simulink model "SF013A_PullCmpActv"  (R2013b)
settings: Solver=FixedStepDiscrete  SolverMode=SingleTasking  StartTime=0.0  StopTime=1  FixedStep=0.002  RelTol=1e-3
values from neighbouring files (symbols this model uses):
  ARCHGLBPRM_100MILLISEC_SEC_F32 = DataDict.Constant    [SF013A_PullCmpActv_DataDict.m]
  ARCHGLBPRM_2MILLISEC_SEC_F32 = DataDict.Constant    [SF013A_PullCmpActv_DataDict.m]
  ARCHGLBPRM_FLOATZEROTHD_ULS_F32 = DataDict.Constant    [SF013A_PullCmpActv_DataDict.m]
  INTGTRSCARSHOTERM_ULS_F32 = DataDict.Constant    [SF013A_PullCmpActv_DataDict.m]
  LONGTERMINTGTRSCAR_ULS_F32 = DataDict.Constant    [SF013A_PullCmpActv_DataDict.m]
  MICROSECTOSEC_ULS_F32 = DataDict.Constant    [SF013A_PullCmpActv_DataDict.m]
  MINSTOSEC_SECPERMINS_F32 = DataDict.Constant    [SF013A_PullCmpActv_DataDict.m]
  PullCmpActvCmpLrnTiDecShoTerm = DataDict.Calibration    [SF013A_PullCmpActv_DataDict.m]
  PullCmpActvCmpLrnTiIncShoTerm = DataDict.Calibration    [SF013A_PullCmpActv_DataDict.m]
  PullCmpActvCmpLrnTiLongTerm = DataDict.Calibration    [SF013A_PullCmpActv_DataDict.m]
  PullCmpActvCmpShoTermRstHwAgThd = DataDict.Calibration    [SF013A_PullCmpActv_DataDict.m]
  PullCmpActvCmpShoTermRstHwTqThd = DataDict.Calibration    [SF013A_PullCmpActv_DataDict.m]
  PullCmpActvCmpShoTermRstLatAThd = DataDict.Calibration    [SF013A_PullCmpActv_DataDict.m]
  PullCmpActvCmpShoTermRstYawRateThd = DataDict.Calibration    [SF013A_PullCmpActv_DataDict.m]
  PullCmpActvEna = DataDict.Calibration    [SF013A_PullCmpActv_DataDict.m]
  PullCmpActvLongTermLim = DataDict.Calibration    [SF013A_PullCmpActv_DataDict.m]
  PullCmpActvLrngEnaAgConfMinMgn = DataDict.Calibration    [SF013A_PullCmpActv_DataDict.m]
  PullCmpActvLrngEnaHwAgMaxMgn = DataDict.Calibration    [SF013A_PullCmpActv_DataDict.m]
  PullCmpActvLrngEnaHwTqMaxMgn = DataDict.Calibration    [SF013A_PullCmpActv_DataDict.m]
  PullCmpActvLrngEnaHwVelMaxMgn = DataDict.Calibration    [SF013A_PullCmpActv_DataDict.m]
  PullCmpActvLrngEnaLatAMaxMgn = DataDict.Calibration    [SF013A_PullCmpActv_DataDict.m]
  PullCmpActvLrngEnaTiThd = DataDict.Calibration    [SF013A_PullCmpActv_DataDict.m]
  PullCmpActvLrngEnaVehSpdMaxMgn = DataDict.Calibration    [SF013A_PullCmpActv_DataDict.m]
  PullCmpActvLrngEnaVehSpdMinMgn = DataDict.Calibration    [SF013A_PullCmpActv_DataDict.m]
  PullCmpActvLrngEnaVehSpdRateMaxMgn = DataDict.Calibration    [SF013A_PullCmpActv_DataDict.m]
  PullCmpActvLrngEnaYawRateMaxMgn = DataDict.Calibration    [SF013A_PullCmpActv_DataDict.m]
  PullCmpActvOpstSignTiShoTerm = DataDict.Calibration    [SF013A_PullCmpActv_DataDict.m]
  PullCmpActvOutpMaxRate = DataDict.Calibration    [SF013A_PullCmpActv_DataDict.m]
  PullCmpActvPullCmpShoTermLim = DataDict.Calibration    [SF013A_PullCmpActv_DataDict.m]
  PullCmpActvPullCmpTotLim = DataDict.Calibration    [SF013A_PullCmpActv_DataDict.m]
  PullCmpActvPullErrLimLongTerm = DataDict.Calibration    [SF013A_PullCmpActv_DataDict.m]
  PullCmpActvPullErrMgnThd = DataDict.Calibration    [SF013A_PullCmpActv_DataDict.m]
  PullCmpActvPullErrShoTermLim = DataDict.Calibration    [SF013A_PullCmpActv_DataDict.m]
  PullCmpActvShoTermRampTi = DataDict.Calibration    [SF013A_PullCmpActv_DataDict.m]
  SysGlbPrmSysTqRat = DataDict.ImprtdCal    [SF013A_PullCmpActv_DataDict.m]
libraries: NxtrAbslt x9, Fil x8, NxtrLim x6, FixdToFloat x3, NxtrSign x3, NxtrMin x3, NxtrNvM x2, NxtrMax x2, simulink x1, FloatToFixd x1, LnrIntrpn x1
(part 2 of 3)

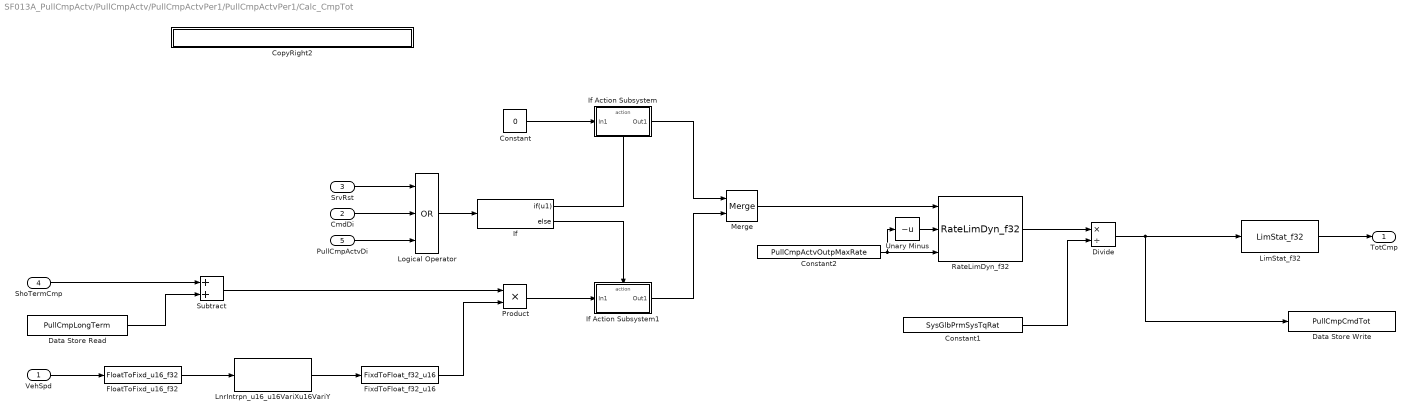
== system SF013A_PullCmpActv/PullCmpActv/PullCmpActvPer1/PullCmpActvPer1/Calc_CmpTot ==
  VehSpd : Inport
  CmdDi : Inport  Port=2
  SrvRst : Inport  Port=3
  ShoTermCmp : Inport  Port=4
  PullCmpActvDi : Inport  Port=5
  Constant : Constant  Value=0  OutDataTypeStr=single
  Constant1 : Constant  Value=SysGlbPrmSysTqRat
  Constant2 : Constant  Value=PullCmpActvOutpMaxRate
  CopyRight2 : Subsystem  Description=|  mask(Copyright Information){none=on}
      | Copyright info block.                                               
      |                                                                     
      | Place copyright information at the top of every subsystem in design.
      mask prompts: none "No parameters"
      mask help: Place copyright information at the top of every subsystem in design.
      mask Display:
      | NxtrConf = 'Nexteer Confidential';
      | 
      | sys = bdroot; %handle for the current model ("system")
      | first = get_param(sys,'Created');
      | if(isempty(first))
      |     first = datestr(now,'yyyy');
      | else
      |     first = first(end-3:end);  %year is last four digits
      | end
      | 
      | last = get_param(sys,'LastModifiedDate');
      | if isempty(last)
      |     last = datestr(now,'yyyy');
      | else
      |     last = last(end-3:end);
      | end
      | 
      | if strcmp(first,last)
      |     fprintf('%s -- Copyright %s Nexteer',NxtrConf,first)
      | else
      |     fprintf('%s -- %s%s- %s Nexteer',NxtrConf,char(169),first,last)
      | end
  Data Store Read : DataStoreRead  DataStoreName=PullCmpLongTerm
  Data Store Write : DataStoreWrite  DataStoreName=PullCmpCmdTot
  Divide : Product  Inputs=*/
  FixdToFloat_f32_u16 : FixdToFloat/FixdToFloat_f32_u16  Param1=14
  FloatToFixd_u16_f32 : FloatToFixd/FloatToFixd_u16_f32  Param1=7
  If : If  IfExpression=u1
  If Action Subsystem : Subsystem  TreatAsAtomicUnit=on
  If Action Subsystem1 : Subsystem  TreatAsAtomicUnit=on
  LimStat_f32 : NxtrLim/LimStat_f32  LoLim=SYSGLBPRM_MOTTQCMDLOLIM_MOTNWTMTR_F32  HiLim=SYSGLBPRM_MOTTQCMDHILIM_MOTNWTMTR_F32
      settings: AttributesFormatString=|
      | Low Limit: %<LoLim>
      | High Limit:%<HiLim>
  LnrIntrpn_u16_u16VariXu16VariY : LnrIntrpn/LnrIntrpn_u16_u16VariXu16VariY  XTbl=PullCmpActvVehSpdScaTblX  YTbl=PullCmpActvVehSpdScaTblY
      settings: AttributesFormatString=Lnr ( u16VariX , u16VariY )
  Logical Operator : Logic  Operator=OR  Inputs=3  AllPortsSameDT=off  OutDataTypeStr=boolean
  Merge : Merge
  Product : Product
  RateLimDyn_f32 : NxtrLim/RateLimDyn_f32  StVar=PullCmpCmdRateLimPrev  Ts=ARCHGLBPRM_2MILLISEC_SEC_F32
      settings: AttributesFormatString=StVar: %<StVar>
  Subtract : Sum
  Unary Minus : UnaryMinus
  TotCmp : Outport
  wires:
  SrvRst/1 -> Logical Operator/1
  CmdDi/1 -> Logical Operator/2
  ShoTermCmp/1 -> Subtract/1
  Data Store Read/1 -> Subtract/2
  FloatToFixd_u16_f32/1 -> LnrIntrpn_u16_u16VariXu16VariY/1
  VehSpd/1 -> FloatToFixd_u16_f32/1
  LnrIntrpn_u16_u16VariXu16VariY/1 -> FixdToFloat_f32_u16/1
  FixdToFloat_f32_u16/1 -> Product/2
  Subtract/1 -> Product/1
  Logical Operator/1 -> If/1
  Constant/1 -> If Action Subsystem/1(In1)
  Product/1 -> If Action Subsystem1/1(In1)
  RateLimDyn_f32/1 -> Divide/1
  Constant1/1 -> Divide/2
  Divide/1 -> Data Store Write/1, LimStat_f32/1
  Merge/1 -> RateLimDyn_f32/1
  If/1 -> If Action Subsystem/Action
  If Action Subsystem/1(Out1) -> Merge/1
  If/2 -> If Action Subsystem1/Action
  If Action Subsystem1/1(Out1) -> Merge/2
  Constant2/1 -> Unary Minus/1, RateLimDyn_f32/3
  Unary Minus/1 -> RateLimDyn_f32/2
  LimStat_f32/1 -> TotCmp/1
  PullCmpActvDi/1 -> Logical Operator/3

== system SF013A_PullCmpActv/PullCmpActv/PullCmpActvPer1/PullCmpActvPer1/CopyRight2 ==

== system SF013A_PullCmpActv/PullCmpActv/PullCmpActvPer1/PullCmpActvPer1/If RstPer1 == True set RstPer1 to False ==
  Action Port : ActionPort  ActionType=then
  Constant : Constant  Value=0  OutDataTypeStr=boolean
  Data Store Write1 : DataStoreWrite  DataStoreName=PullCmpShoTermRst
  wires:
  Constant/1 -> Data Store Write1/1

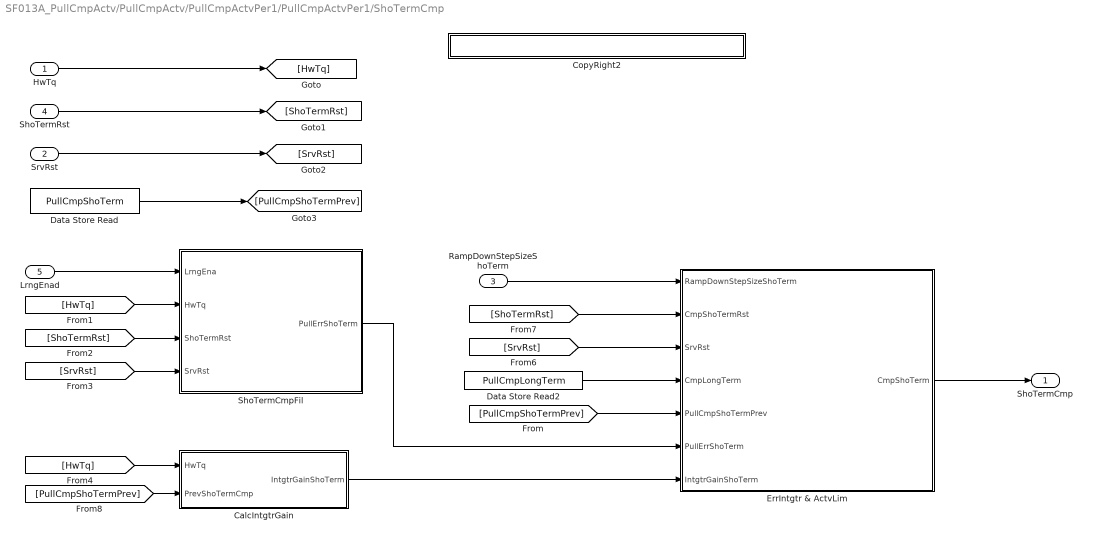
== system SF013A_PullCmpActv/PullCmpActv/PullCmpActvPer1/PullCmpActvPer1/ShoTermCmp ==
  "HwTq " : Inport
  SrvRst : Inport  Port=2
  RampDownStepSizeShoTerm : Inport  Port=3
  ShoTermRst : Inport  Port=4
  LrngEnad : Inport  Port=5
  "CalcIntgtrGain " : Subsystem  TreatAsAtomicUnit=on
  CopyRight2 : Subsystem  Description=|  mask(Copyright Information){none=on}
      | Copyright info block.                                               
      |                                                                     
      | Place copyright information at the top of every subsystem in design.
      mask prompts: none "No parameters"
      mask help: Place copyright information at the top of every subsystem in design.
      mask Display:
      | NxtrConf = 'Nexteer Confidential';
      | 
      | sys = bdroot; %handle for the current model ("system")
      | first = get_param(sys,'Created');
      | if(isempty(first))
      |     first = datestr(now,'yyyy');
      | else
      |     first = first(end-3:end);  %year is last four digits
      | end
      | 
      | last = get_param(sys,'LastModifiedDate');
      | if isempty(last)
      |     last = datestr(now,'yyyy');
      | else
      |     last = last(end-3:end);
      | end
      | 
      | if strcmp(first,last)
      |     fprintf('%s -- Copyright %s Nexteer',NxtrConf,first)
      | else
      |     fprintf('%s -- %s%s- %s Nexteer',NxtrConf,char(169),first,last)
      | end
  Data Store Read : DataStoreRead  DataStoreName=PullCmpShoTerm
  Data Store Read2 : DataStoreRead  DataStoreName=PullCmpLongTerm
  "ErrIntgtr & ActvLim " : Subsystem  TreatAsAtomicUnit=on
  ShoTermCmpFil : Subsystem  TreatAsAtomicUnit=on
  ShoTermCmp : Outport
  wires:
  "HwTq "/1 -> [HwTq]
  ShoTermRst/1 -> [ShoTermRst]
  SrvRst/1 -> [SrvRst]
  ShoTermCmpFil/1(PullErrShoTerm) -> "ErrIntgtr & ActvLim "/6(PullErrShoTerm)
  [HwTq] -> ShoTermCmpFil/2("HwTq ")
  LrngEnad/1 -> ShoTermCmpFil/1(LrngEna)
  [ShoTermRst] -> ShoTermCmpFil/3(ShoTermRst)
  [SrvRst] -> ShoTermCmpFil/4(SrvRst)
  [HwTq] -> "CalcIntgtrGain "/1("HwTq ")
  [PullCmpShoTermPrev] -> "CalcIntgtrGain "/2(PrevShoTermCmp)
  "CalcIntgtrGain "/1(IntgtrGainShoTerm) -> "ErrIntgtr & ActvLim "/7(IntgtrGainShoTerm)
  Data Store Read2/1 -> "ErrIntgtr & ActvLim "/4(CmpLongTerm)
  [PullCmpShoTermPrev] -> "ErrIntgtr & ActvLim "/5(PullCmpShoTermPrev)
  [SrvRst] -> "ErrIntgtr & ActvLim "/3("SrvRst ")
  [ShoTermRst] -> "ErrIntgtr & ActvLim "/2("CmpShoTermRst ")
  "ErrIntgtr & ActvLim "/1("CmpShoTerm ") -> ShoTermCmp/1
  Data Store Read/1 -> [PullCmpShoTermPrev]
  RampDownStepSizeShoTerm/1 -> "ErrIntgtr & ActvLim "/1(RampDownStepSizeShoTerm)

== system SF013A_PullCmpActv/PullCmpActv/PullCmpActvPer2/PullCmpActvPer2/CopyRight2 ==

== system SF013A_PullCmpActv/PullCmpActv/PullCmpActvPer2/PullCmpActvPer2/If PullCmpLongTermRst == True set PullCmpLongTermRst to False ==
  Action Port : ActionPort  ActionType=then
  Constant : Constant  Value=0  OutDataTypeStr=boolean
  CopyRight2 : Subsystem  Description=|  mask(Copyright Information){none=on}
      | Copyright info block.                                               
      |                                                                     
      | Place copyright information at the top of every subsystem in design.
      mask prompts: none "No parameters"
      mask help: Place copyright information at the top of every subsystem in design.
      mask Display:
      | NxtrConf = 'Nexteer Confidential';
      | 
      | sys = bdroot; %handle for the current model ("system")
      | first = get_param(sys,'Created');
      | if(isempty(first))
      |     first = datestr(now,'yyyy');
      | else
      |     first = first(end-3:end);  %year is last four digits
      | end
      | 
      | last = get_param(sys,'LastModifiedDate');
      | if isempty(last)
      |     last = datestr(now,'yyyy');
      | else
      |     last = last(end-3:end);
      | end
      | 
      | if strcmp(first,last)
      |     fprintf('%s -- Copyright %s Nexteer',NxtrConf,first)
      | else
      |     fprintf('%s -- %s%s- %s Nexteer',NxtrConf,char(169),first,last)
      | end
  Data Store Write1 : DataStoreWrite  DataStoreName=PullCmpLongTermRst
  wires:
  Constant/1 -> Data Store Write1/1

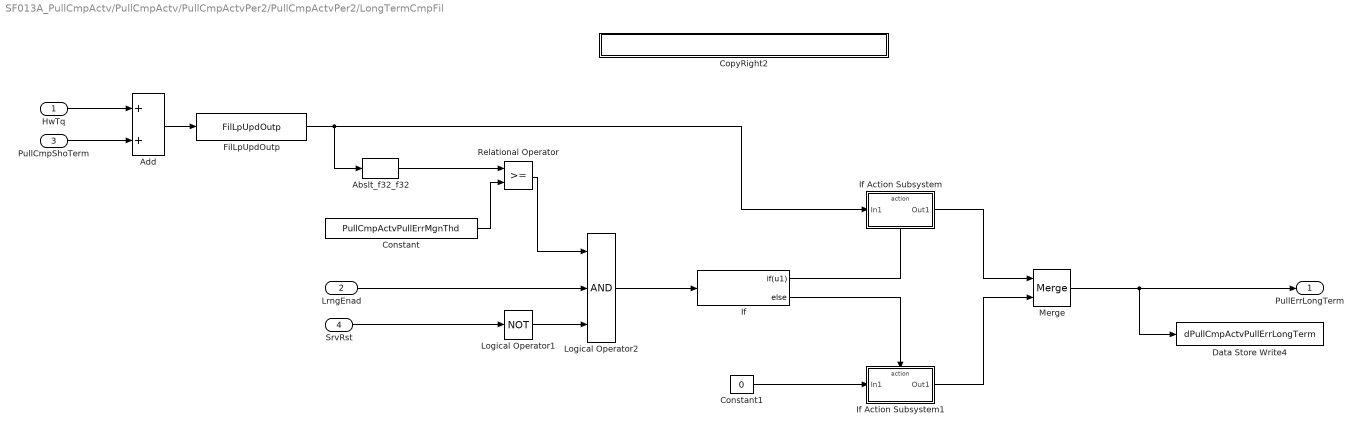
== system SF013A_PullCmpActv/PullCmpActv/PullCmpActvPer2/PullCmpActvPer2/LongTermCmpFil ==
  "HwTq " : Inport
  LrngEnad : Inport  Port=2
  PullCmpShoTerm : Inport  Port=3
  SrvRst : Inport  Port=4
  Abslt_f32_f32 : NxtrAbslt/Abslt_f32_f32  SFunctionSpec=single y1 = Abslt_f32_f32(single u1)
      settings: AttributesFormatString=%<Name>
  Add : Sum
  Constant : Constant  Value=PullCmpActvPullErrMgnThd
  Constant1 : Constant  Value=0  OutDataTypeStr=single
  CopyRight2 : Subsystem  Description=|  mask(Copyright Information){none=on}
      | Copyright info block.                                               
      |                                                                     
      | Place copyright information at the top of every subsystem in design.
      mask prompts: none "No parameters"
      mask help: Place copyright information at the top of every subsystem in design.
      mask Display:
      | NxtrConf = 'Nexteer Confidential';
      | 
      | sys = bdroot; %handle for the current model ("system")
      | first = get_param(sys,'Created');
      | if(isempty(first))
      |     first = datestr(now,'yyyy');
      | else
      |     first = first(end-3:end);  %year is last four digits
      | end
      | 
      | last = get_param(sys,'LastModifiedDate');
      | if isempty(last)
      |     last = datestr(now,'yyyy');
      | else
      |     last = last(end-3:end);
      | end
      | 
      | if strcmp(first,last)
      |     fprintf('%s -- Copyright %s Nexteer',NxtrConf,first)
      | else
      |     fprintf('%s -- %s%s- %s Nexteer',NxtrConf,char(169),first,last)
      | end
  Data Store Write4 : DataStoreWrite  DataStoreName=dPullCmpActvPullErrLongTerm
  FilLpUpdOutp : Fil/FilLpUpdOutp  StVar=HwTqLpFilLongTerm
      settings: AttributesFormatString=StVar: %<StVar>
  If : If  IfExpression=u1
  If Action Subsystem : Subsystem  TreatAsAtomicUnit=on
  If Action Subsystem1 : Subsystem  TreatAsAtomicUnit=on
  Logical Operator1 : Logic  Operator=NOT  Inputs=1  AllPortsSameDT=off  OutDataTypeStr=boolean
  Logical Operator2 : Logic  Inputs=3  AllPortsSameDT=off  OutDataTypeStr=boolean
  Merge : Merge
  Relational Operator : RelationalOperator  OutDataTypeStr=boolean
  PullErrLongTerm : Outport
  wires:
  FilLpUpdOutp/1 -> Abslt_f32_f32/1, If Action Subsystem/1(In1)
  Abslt_f32_f32/1 -> Relational Operator/1
  Constant/1 -> Relational Operator/2
  SrvRst/1 -> Logical Operator1/1
  Relational Operator/1 -> Logical Operator2/1
  LrngEnad/1 -> Logical Operator2/2
  Logical Operator1/1 -> Logical Operator2/3
  Constant1/1 -> If Action Subsystem1/1(In1)
  Merge/1 -> Data Store Write4/1, PullErrLongTerm/1
  Add/1 -> FilLpUpdOutp/1
  "HwTq "/1 -> Add/1
  PullCmpShoTerm/1 -> Add/2
  Logical Operator2/1 -> If/1
  If/1 -> If Action Subsystem/Action
  If/2 -> If Action Subsystem1/Action
  If Action Subsystem/1(Out1) -> Merge/1
  If Action Subsystem1/1(Out1) -> Merge/2

== system SF013A_PullCmpActv/PullCmpActv/PullCmpActvPer2/PullCmpActvPer2/LongTermErrIntgtr  ==
  "SrvRst " : Inport
  CmpLongTermPrev : Inport  Port=2
  PullErrLongTerm : Inport  Port=3
  Constant1 : Constant  Value=0  OutDataTypeStr=single
  CopyRight2 : Subsystem  Description=|  mask(Copyright Information){none=on}
      | Copyright info block.                                               
      |                                                                     
      | Place copyright information at the top of every subsystem in design.
      mask prompts: none "No parameters"
      mask help: Place copyright information at the top of every subsystem in design.
      mask Display:
      | NxtrConf = 'Nexteer Confidential';
      | 
      | sys = bdroot; %handle for the current model ("system")
      | first = get_param(sys,'Created');
      | if(isempty(first))
      |     first = datestr(now,'yyyy');
      | else
      |     first = first(end-3:end);  %year is last four digits
      | end
      | 
      | last = get_param(sys,'LastModifiedDate');
      | if isempty(last)
      |     last = datestr(now,'yyyy');
      | else
      |     last = last(end-3:end);
      | end
      | 
      | if strcmp(first,last)
      |     fprintf('%s -- Copyright %s Nexteer',NxtrConf,first)
      | else
      |     fprintf('%s -- %s%s- %s Nexteer',NxtrConf,char(169),first,last)
      | end
  Data Store Write2 : DataStoreWrite  DataStoreName=PullCmpLongTerm
  If : If  IfExpression=u1
  If Action Subsystem : Subsystem  TreatAsAtomicUnit=on
  If Action Subsystem1 : Subsystem  TreatAsAtomicUnit=on
  Merge : Merge
  wires:
  "SrvRst "/1 -> If/1
  Constant1/1 -> If Action Subsystem/1(In1)
  If/1 -> If Action Subsystem/Action
  If/2 -> If Action Subsystem1/Action
  Merge/1 -> Data Store Write2/1
  If Action Subsystem/1(Out1) -> Merge/1
  If Action Subsystem1/1(CmpLongTerm) -> Merge/2
  PullErrLongTerm/1 -> If Action Subsystem1/1(PullErrLongTerm)
  CmpLongTermPrev/1 -> If Action Subsystem1/2(CmpLongTermPrev)

== system SF013A_PullCmpActv/PullCmpActv/PullCmpActvPer1/PullCmpActvPer1/ActvCmpEna/CopyRight2 ==

== system SF013A_PullCmpActv/PullCmpActv/PullCmpActvPer1/PullCmpActvPer1/ActvCmpEna/ElapsedTime ==
  LrngEna : Inport
  Data Store Read : DataStoreRead  Priority=1  DataStoreName=LrngEnaPrev
      settings: AttributesFormatString="priority:  %<Priority>"
  Data Store Write : DataStoreWrite  Priority=2  DataStoreName=LrngEnaPrev
      settings: AttributesFormatString="priority:  %<Priority>"
  If : If  NumInputs=2  IfExpression=u1  ElseIfExpressions=u2
  If not true elapsed time = 0 : Subsystem  TreatAsAtomicUnit=on
  "If true and last step is true calculate elapsed time " : Subsystem  TreatAsAtomicUnit=on
  "If true and last step not true elapsed time = 0 get reference time " : Subsystem  TreatAsAtomicUnit=on
  Logical Operator : Logic  AllPortsSameDT=off  OutDataTypeStr=boolean
  Logical Operator1 : Logic  Operator=NOT  AllPortsSameDT=off  OutDataTypeStr=boolean
  Logical Operator2 : Logic  Operator=NOT  AllPortsSameDT=off  OutDataTypeStr=boolean
  Merge : Merge  Inputs=3
  ElapsedTime : Outport
  wires:
  If/1 -> If not true elapsed time = 0/Action
  If/2 -> "If true and last step not true elapsed time = 0 get reference time "/Action
  If/3 -> "If true and last step is true calculate elapsed time "/Action
  If not true elapsed time = 0/1(SpanTi) -> Merge/1
  "If true and last step not true elapsed time = 0 get reference time "/1("SpanTi ") -> Merge/2
  "If true and last step is true calculate elapsed time "/1(SpanTi) -> Merge/3
  Merge/1 -> ElapsedTime/1
  LrngEna/1 -> Logical Operator/1, Logical Operator2/1, Data Store Write/1
  Logical Operator1/1 -> Logical Operator/2
  Data Store Read/1 -> Logical Operator1/1
  Logical Operator/1 -> If/2
  Logical Operator2/1 -> If/1

== system SF013A_PullCmpActv/PullCmpActv/PullCmpActvPer1/PullCmpActvPer1/Calc_CmpTot/CopyRight2 ==

== system SF013A_PullCmpActv/PullCmpActv/PullCmpActvPer1/PullCmpActvPer1/Calc_CmpTot/If Action Subsystem ==
  In1 : Inport
  Action Port : ActionPort  ActionType=then
  CopyRight2 : Subsystem  Description=|  mask(Copyright Information){none=on}
      | Copyright info block.                                               
      |                                                                     
      | Place copyright information at the top of every subsystem in design.
      mask prompts: none "No parameters"
      mask help: Place copyright information at the top of every subsystem in design.
      mask Display:
      | NxtrConf = 'Nexteer Confidential';
      | 
      | sys = bdroot; %handle for the current model ("system")
      | first = get_param(sys,'Created');
      | if(isempty(first))
      |     first = datestr(now,'yyyy');
      | else
      |     first = first(end-3:end);  %year is last four digits
      | end
      | 
      | last = get_param(sys,'LastModifiedDate');
      | if isempty(last)
      |     last = datestr(now,'yyyy');
      | else
      |     last = last(end-3:end);
      | end
      | 
      | if strcmp(first,last)
      |     fprintf('%s -- Copyright %s Nexteer',NxtrConf,first)
      | else
      |     fprintf('%s -- %s%s- %s Nexteer',NxtrConf,char(169),first,last)
      | end
  Out1 : Outport
  wires:
  In1/1 -> Out1/1

== system SF013A_PullCmpActv/PullCmpActv/PullCmpActvPer1/PullCmpActvPer1/Calc_CmpTot/If Action Subsystem1 ==
  In1 : Inport
  Action Port : ActionPort  ActionType=else
  CopyRight2 : Subsystem  Description=|  mask(Copyright Information){none=on}
      | Copyright info block.                                               
      |                                                                     
      | Place copyright information at the top of every subsystem in design.
      mask prompts: none "No parameters"
      mask help: Place copyright information at the top of every subsystem in design.
      mask Display:
      | NxtrConf = 'Nexteer Confidential';
      | 
      | sys = bdroot; %handle for the current model ("system")
      | first = get_param(sys,'Created');
      | if(isempty(first))
      |     first = datestr(now,'yyyy');
      | else
      |     first = first(end-3:end);  %year is last four digits
      | end
      | 
      | last = get_param(sys,'LastModifiedDate');
      | if isempty(last)
      |     last = datestr(now,'yyyy');
      | else
      |     last = last(end-3:end);
      | end
      | 
      | if strcmp(first,last)
      |     fprintf('%s -- Copyright %s Nexteer',NxtrConf,first)
      | else
      |     fprintf('%s -- %s%s- %s Nexteer',NxtrConf,char(169),first,last)
      | end
  Out1 : Outport
  wires:
  In1/1 -> Out1/1

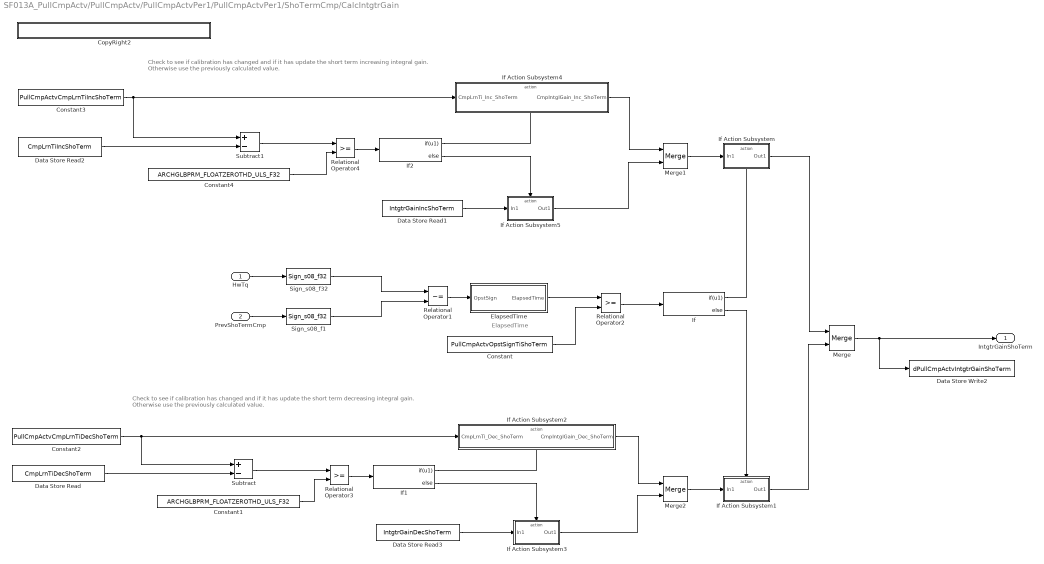
== system SF013A_PullCmpActv/PullCmpActv/PullCmpActvPer1/PullCmpActvPer1/ShoTermCmp/CalcIntgtrGain  ==
  note: Check to see if calibration has changed and if it has update the short term increasing integral gain.
      | Otherwise use the previously calculated value.
  note: ElapsedTime
  note: Check to see if calibration has changed and if it has update the short term decreasing integral gain.
      | Otherwise use the previously calculated value.
  "HwTq " : Inport
  PrevShoTermCmp : Inport  Port=2
  Constant : Constant  Value=PullCmpActvOpstSignTiShoTerm
  Constant1 : Constant  Value=ARCHGLBPRM_FLOATZEROTHD_ULS_F32
  Constant2 : Constant  Value=PullCmpActvCmpLrnTiDecShoTerm
  Constant3 : Constant  Value=PullCmpActvCmpLrnTiIncShoTerm
  Constant4 : Constant  Value=ARCHGLBPRM_FLOATZEROTHD_ULS_F32
  CopyRight2 : Subsystem  Description=|  mask(Copyright Information){none=on}
      | Copyright info block.                                               
      |                                                                     
      | Place copyright information at the top of every subsystem in design.
      mask prompts: none "No parameters"
      mask help: Place copyright information at the top of every subsystem in design.
      mask Display:
      | NxtrConf = 'Nexteer Confidential';
      | 
      | sys = bdroot; %handle for the current model ("system")
      | first = get_param(sys,'Created');
      | if(isempty(first))
      |     first = datestr(now,'yyyy');
      | else
      |     first = first(end-3:end);  %year is last four digits
      | end
      | 
      | last = get_param(sys,'LastModifiedDate');
      | if isempty(last)
      |     last = datestr(now,'yyyy');
      | else
      |     last = last(end-3:end);
      | end
      | 
      | if strcmp(first,last)
      |     fprintf('%s -- Copyright %s Nexteer',NxtrConf,first)
      | else
      |     fprintf('%s -- %s%s- %s Nexteer',NxtrConf,char(169),first,last)
      | end
  Data Store Read : DataStoreRead  DataStoreName=CmpLrnTiDecShoTerm
  Data Store Read1 : DataStoreRead  DataStoreName=IntgtrGainIncShoTerm
  Data Store Read2 : DataStoreRead  DataStoreName=CmpLrnTiIncShoTerm
  Data Store Read3 : DataStoreRead  DataStoreName=IntgtrGainDecShoTerm
  Data Store Write2 : DataStoreWrite  DataStoreName=dPullCmpActvIntgtrGainShoTerm
  ElapsedTime : Subsystem  TreatAsAtomicUnit=on
  If : If  IfExpression=u1
  If Action Subsystem : Subsystem  TreatAsAtomicUnit=on
  If Action Subsystem1 : Subsystem  TreatAsAtomicUnit=on
  If Action Subsystem2 : Subsystem  TreatAsAtomicUnit=on
  If Action Subsystem3 : Subsystem  TreatAsAtomicUnit=on
  If Action Subsystem4 : Subsystem  TreatAsAtomicUnit=on
  If Action Subsystem5 : Subsystem  TreatAsAtomicUnit=on
  If1 : If  IfExpression=u1
  If2 : If  IfExpression=u1
  Merge : Merge
  Merge1 : Merge
  Merge2 : Merge
  Relational Operator1 : RelationalOperator  Operator=~=  OutDataTypeStr=boolean
  Relational Operator2 : RelationalOperator  OutDataTypeStr=boolean
  Relational Operator3 : RelationalOperator  OutDataTypeStr=boolean
  Relational Operator4 : RelationalOperator  OutDataTypeStr=boolean
  Sign_s08_f1 : NxtrSign/Sign_s08_f32  SFunctionSpec=int8 y1 = Sign_s08_f32(single u1)
  Sign_s08_f32 : NxtrSign/Sign_s08_f32  SFunctionSpec=int8 y1 = Sign_s08_f32(single u1)
  Subtract : Sum  Inputs=+-
  Subtract1 : Sum  Inputs=+-
  IntgtrGainShoTerm : Outport
  wires:
  Relational Operator3/1 -> If1/1
  Data Store Read/1 -> Subtract/2
  If1/1 -> If Action Subsystem2/Action
  Constant2/1 -> Subtract/1, If Action Subsystem2/1(CmpLrnTi_Dec_ShoTerm)
  If2/1 -> If Action Subsystem4/Action
  Relational Operator4/1 -> If2/1
  Subtract/1 -> Relational Operator3/1
  Constant1/1 -> Relational Operator3/2
  Data Store Read2/1 -> Subtract1/2
  Constant3/1 -> If Action Subsystem4/1(CmpLrnTi_Inc_ShoTerm), Subtract1/1
  Subtract1/1 -> Relational Operator4/1
  Constant4/1 -> Relational Operator4/2
  "HwTq "/1 -> Sign_s08_f32/1
  PrevShoTermCmp/1 -> Sign_s08_f1/1
  Relational Operator1/1 -> ElapsedTime/1("OpstSign ")
  ElapsedTime/1(ElapsedTime) -> Relational Operator2/1
  Constant/1 -> Relational Operator2/2
  Merge/1 -> IntgtrGainShoTerm/1, Data Store Write2/1
  If/1 -> If Action Subsystem/Action
  If/2 -> If Action Subsystem1/Action
  Relational Operator2/1 -> If/1
  If Action Subsystem/1(Out1) -> Merge/1
  If Action Subsystem1/1(Out1) -> Merge/2
  Sign_s08_f32/1 -> Relational Operator1/1
  Sign_s08_f1/1 -> Relational Operator1/2
  If2/2 -> If Action Subsystem5/Action
  Data Store Read1/1 -> If Action Subsystem5/1(In1)
  If Action Subsystem5/1(Out1) -> Merge1/2
  If1/2 -> If Action Subsystem3/Action
  Data Store Read3/1 -> If Action Subsystem3/1(In1)
  If Action Subsystem4/1(CmpIntglGain_Inc_ShoTerm) -> Merge1/1
  Merge1/1 -> If Action Subsystem/1(In1)
  Merge2/1 -> If Action Subsystem1/1(In1)
  If Action Subsystem3/1(Out1) -> Merge2/2
  If Action Subsystem2/1(CmpIntglGain_Dec_ShoTerm) -> Merge2/1

== system SF013A_PullCmpActv/PullCmpActv/PullCmpActvPer1/PullCmpActvPer1/ShoTermCmp/CopyRight2 ==

== system SF013A_PullCmpActv/PullCmpActv/PullCmpActvPer1/PullCmpActvPer1/ShoTermCmp/ErrIntgtr & ActvLim  ==
  RampDownStepSizeShoTerm : Inport
  "CmpShoTermRst " : Inport  Port=2
  "SrvRst " : Inport  Port=3
  CmpLongTerm : Inport  Port=4
  PullCmpShoTermPrev : Inport  Port=5
  PullErrShoTerm : Inport  Port=6
  IntgtrGainShoTerm : Inport  Port=7
  Constant8 : Constant  Value=0  OutDataTypeStr=single
  CopyRight2 : Subsystem  Description=|  mask(Copyright Information){none=on}
      | Copyright info block.                                               
      |                                                                     
      | Place copyright information at the top of every subsystem in design.
      mask prompts: none "No parameters"
      mask help: Place copyright information at the top of every subsystem in design.
      mask Display:
      | NxtrConf = 'Nexteer Confidential';
      | 
      | sys = bdroot; %handle for the current model ("system")
      | first = get_param(sys,'Created');
      | if(isempty(first))
      |     first = datestr(now,'yyyy');
      | else
      |     first = first(end-3:end);  %year is last four digits
      | end
      | 
      | last = get_param(sys,'LastModifiedDate');
      | if isempty(last)
      |     last = datestr(now,'yyyy');
      | else
      |     last = last(end-3:end);
      | end
      | 
      | if strcmp(first,last)
      |     fprintf('%s -- Copyright %s Nexteer',NxtrConf,first)
      | else
      |     fprintf('%s -- %s%s- %s Nexteer',NxtrConf,char(169),first,last)
      | end
  Data Store Write : DataStoreWrite  DataStoreName=PullCmpShoTerm
  If Action Subsystem2 : Subsystem  TreatAsAtomicUnit=on
  If Action Subsystem3 : Subsystem  TreatAsAtomicUnit=on
  If1 : If  IfExpression=u1
  Merge : Merge
  "CmpShoTerm " : Outport
  wires:
  "CmpShoTermRst "/1 -> If Action Subsystem3/2("CmpShoTermRst ")
  RampDownStepSizeShoTerm/1 -> If Action Subsystem3/5(RampDownStepSizeShoTerm)
  If1/1 -> If Action Subsystem2/Action
  If1/2 -> If Action Subsystem3/Action
  PullErrShoTerm/1 -> If Action Subsystem3/1(PullErrShoTerm)
  CmpLongTerm/1 -> If Action Subsystem3/3(CmpLongTerm)
  IntgtrGainShoTerm/1 -> If Action Subsystem3/4(IntgtrGainShoTerm)
  Constant8/1 -> If Action Subsystem2/1(In1)
  "SrvRst "/1 -> If1/1
  If Action Subsystem2/1(Out1) -> Merge/1
  If Action Subsystem3/1(PullCmpShoTerm) -> Merge/2
  Merge/1 -> Data Store Write/1, "CmpShoTerm "/1
  PullCmpShoTermPrev/1 -> If Action Subsystem3/6(PullCmpShoTermPrev)

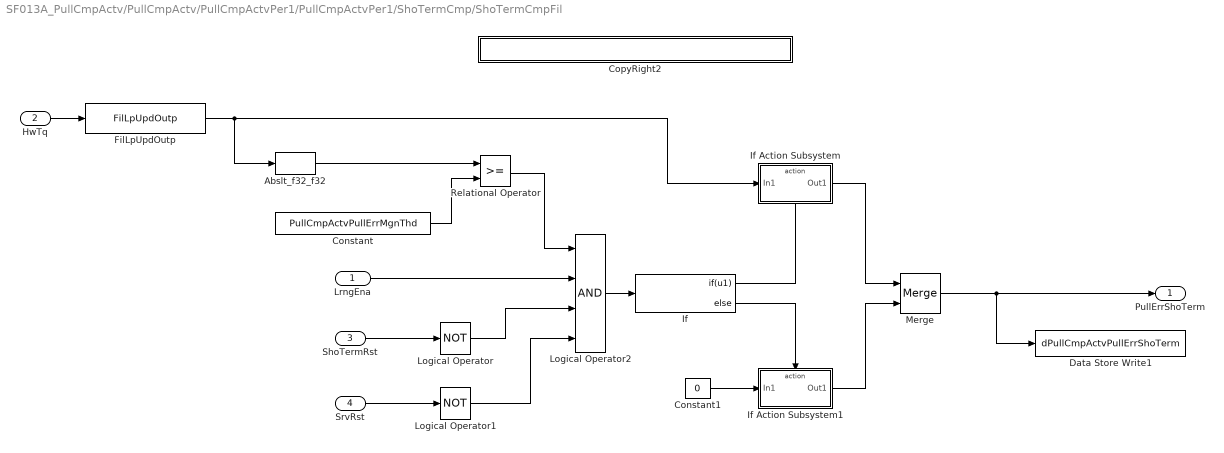
== system SF013A_PullCmpActv/PullCmpActv/PullCmpActvPer1/PullCmpActvPer1/ShoTermCmp/ShoTermCmpFil ==
  LrngEna : Inport
  "HwTq " : Inport  Port=2
  ShoTermRst : Inport  Port=3
  SrvRst : Inport  Port=4
  Abslt_f32_f32 : NxtrAbslt/Abslt_f32_f32  SFunctionSpec=single y1 = Abslt_f32_f32(single u1)
      settings: AttributesFormatString=%<Name>
  Constant : Constant  Value=PullCmpActvPullErrMgnThd
  Constant1 : Constant  Value=0  OutDataTypeStr=single
  CopyRight2 : Subsystem  Description=|  mask(Copyright Information){none=on}
      | Copyright info block.                                               
      |                                                                     
      | Place copyright information at the top of every subsystem in design.
      mask prompts: none "No parameters"
      mask help: Place copyright information at the top of every subsystem in design.
      mask Display:
      | NxtrConf = 'Nexteer Confidential';
      | 
      | sys = bdroot; %handle for the current model ("system")
      | first = get_param(sys,'Created');
      | if(isempty(first))
      |     first = datestr(now,'yyyy');
      | else
      |     first = first(end-3:end);  %year is last four digits
      | end
      | 
      | last = get_param(sys,'LastModifiedDate');
      | if isempty(last)
      |     last = datestr(now,'yyyy');
      | else
      |     last = last(end-3:end);
      | end
      | 
      | if strcmp(first,last)
      |     fprintf('%s -- Copyright %s Nexteer',NxtrConf,first)
      | else
      |     fprintf('%s -- %s%s- %s Nexteer',NxtrConf,char(169),first,last)
      | end
  Data Store Write1 : DataStoreWrite  DataStoreName=dPullCmpActvPullErrShoTerm
  FilLpUpdOutp : Fil/FilLpUpdOutp  StVar=HwTqLpFilShoTerm
      settings: AttributesFormatString=StVar: %<StVar>
  If : If  IfExpression=u1
  If Action Subsystem : Subsystem  TreatAsAtomicUnit=on
  If Action Subsystem1 : Subsystem  TreatAsAtomicUnit=on
  Logical Operator : Logic  Operator=NOT  Inputs=1  AllPortsSameDT=off  OutDataTypeStr=boolean
  Logical Operator1 : Logic  Operator=NOT  Inputs=1  AllPortsSameDT=off  OutDataTypeStr=boolean
  Logical Operator2 : Logic  Inputs=4  AllPortsSameDT=off  OutDataTypeStr=boolean
  Merge : Merge
  Relational Operator : RelationalOperator  OutDataTypeStr=boolean
  PullErrShoTerm : Outport
  wires:
  "HwTq "/1 -> FilLpUpdOutp/1
  FilLpUpdOutp/1 -> If Action Subsystem/1(In1), Abslt_f32_f32/1
  Abslt_f32_f32/1 -> Relational Operator/1
  Constant/1 -> Relational Operator/2
  SrvRst/1 -> Logical Operator1/1
  ShoTermRst/1 -> Logical Operator/1
  Relational Operator/1 -> Logical Operator2/1
  LrngEna/1 -> Logical Operator2/2
  Logical Operator/1 -> Logical Operator2/3
  Logical Operator1/1 -> Logical Operator2/4
  Logical Operator2/1 -> If/1
  Constant1/1 -> If Action Subsystem1/1(In1)
  Merge/1 -> Data Store Write1/1, PullErrShoTerm/1
  If/1 -> If Action Subsystem/Action
  If/2 -> If Action Subsystem1/Action
  If Action Subsystem/1(Out1) -> Merge/1
  If Action Subsystem1/1(Out1) -> Merge/2

== system SF013A_PullCmpActv/PullCmpActv/PullCmpActvPer2/PullCmpActvPer2/If PullCmpLongTermRst == True set PullCmpLongTermRst to False/CopyRight2 ==

== system SF013A_PullCmpActv/PullCmpActv/PullCmpActvPer2/PullCmpActvPer2/LongTermCmpFil/CopyRight2 ==

== system SF013A_PullCmpActv/PullCmpActv/PullCmpActvPer2/PullCmpActvPer2/LongTermCmpFil/If Action Subsystem ==
  In1 : Inport
  Action Port : ActionPort  ActionType=then
  CopyRight2 : Subsystem  Description=|  mask(Copyright Information){none=on}
      | Copyright info block.                                               
      |                                                                     
      | Place copyright information at the top of every subsystem in design.
      mask prompts: none "No parameters"
      mask help: Place copyright information at the top of every subsystem in design.
      mask Display:
      | NxtrConf = 'Nexteer Confidential';
      | 
      | sys = bdroot; %handle for the current model ("system")
      | first = get_param(sys,'Created');
      | if(isempty(first))
      |     first = datestr(now,'yyyy');
      | else
      |     first = first(end-3:end);  %year is last four digits
      | end
      | 
      | last = get_param(sys,'LastModifiedDate');
      | if isempty(last)
      |     last = datestr(now,'yyyy');
      | else
      |     last = last(end-3:end);
      | end
      | 
      | if strcmp(first,last)
      |     fprintf('%s -- Copyright %s Nexteer',NxtrConf,first)
      | else
      |     fprintf('%s -- %s%s- %s Nexteer',NxtrConf,char(169),first,last)
      | end
  Out1 : Outport
  wires:
  In1/1 -> Out1/1

== system SF013A_PullCmpActv/PullCmpActv/PullCmpActvPer2/PullCmpActvPer2/LongTermCmpFil/If Action Subsystem1 ==
  In1 : Inport
  Action Port : ActionPort  ActionType=else
  CopyRight2 : Subsystem  Description=|  mask(Copyright Information){none=on}
      | Copyright info block.                                               
      |                                                                     
      | Place copyright information at the top of every subsystem in design.
      mask prompts: none "No parameters"
      mask help: Place copyright information at the top of every subsystem in design.
      mask Display:
      | NxtrConf = 'Nexteer Confidential';
      | 
      | sys = bdroot; %handle for the current model ("system")
      | first = get_param(sys,'Created');
      | if(isempty(first))
      |     first = datestr(now,'yyyy');
      | else
      |     first = first(end-3:end);  %year is last four digits
      | end
      | 
      | last = get_param(sys,'LastModifiedDate');
      | if isempty(last)
      |     last = datestr(now,'yyyy');
      | else
      |     last = last(end-3:end);
      | end
      | 
      | if strcmp(first,last)
      |     fprintf('%s -- Copyright %s Nexteer',NxtrConf,first)
      | else
      |     fprintf('%s -- %s%s- %s Nexteer',NxtrConf,char(169),first,last)
      | end
  Out1 : Outport
  wires:
  In1/1 -> Out1/1

== system SF013A_PullCmpActv/PullCmpActv/PullCmpActvPer2/PullCmpActvPer2/LongTermErrIntgtr /CopyRight2 ==

== system SF013A_PullCmpActv/PullCmpActv/PullCmpActvPer2/PullCmpActvPer2/LongTermErrIntgtr /If Action Subsystem ==
  In1 : Inport
  Action Port : ActionPort  ActionType=then
  CopyRight2 : Subsystem  Description=|  mask(Copyright Information){none=on}
      | Copyright info block.                                               
      |                                                                     
      | Place copyright information at the top of every subsystem in design.
      mask prompts: none "No parameters"
      mask help: Place copyright information at the top of every subsystem in design.
      mask Display:
      | NxtrConf = 'Nexteer Confidential';
      | 
      | sys = bdroot; %handle for the current model ("system")
      | first = get_param(sys,'Created');
      | if(isempty(first))
      |     first = datestr(now,'yyyy');
      | else
      |     first = first(end-3:end);  %year is last four digits
      | end
      | 
      | last = get_param(sys,'LastModifiedDate');
      | if isempty(last)
      |     last = datestr(now,'yyyy');
      | else
      |     last = last(end-3:end);
      | end
      | 
      | if strcmp(first,last)
      |     fprintf('%s -- Copyright %s Nexteer',NxtrConf,first)
      | else
      |     fprintf('%s -- %s%s- %s Nexteer',NxtrConf,char(169),first,last)
      | end
  Out1 : Outport
  wires:
  In1/1 -> Out1/1

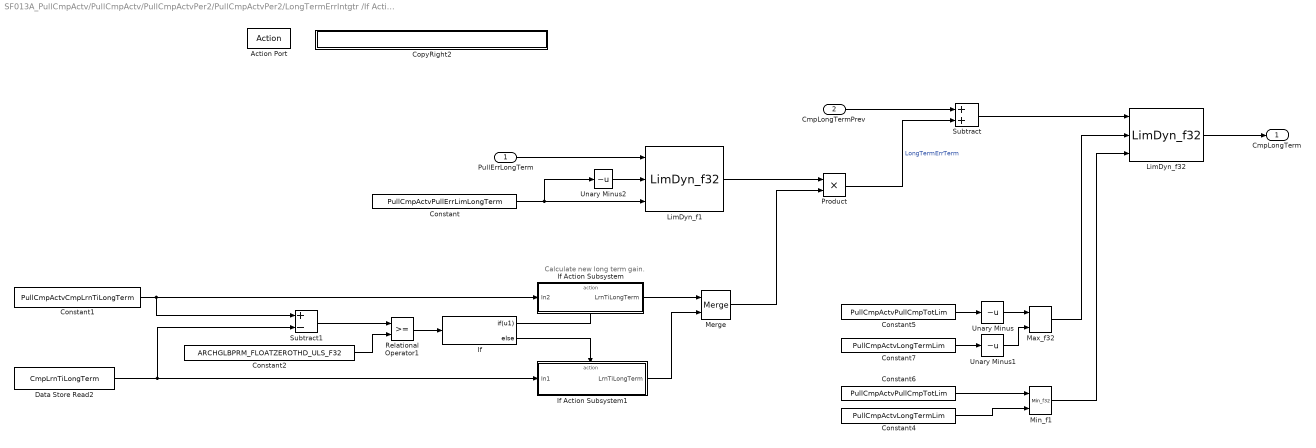
== system SF013A_PullCmpActv/PullCmpActv/PullCmpActvPer2/PullCmpActvPer2/LongTermErrIntgtr /If Action Subsystem1 ==
  note: Calculate new long term gain.
  PullErrLongTerm : Inport
  CmpLongTermPrev : Inport  Port=2
  Action Port : ActionPort  ActionType=else
  Constant : Constant  Value=PullCmpActvPullErrLimLongTerm
  Constant1 : Constant  Value=PullCmpActvCmpLrnTiLongTerm
  Constant2 : Constant  Value=ARCHGLBPRM_FLOATZEROTHD_ULS_F32
  Constant4 : Constant  Value=PullCmpActvLongTermLim
  Constant5 : Constant  Value=PullCmpActvPullCmpTotLim
  Constant6 : Constant  Value=PullCmpActvPullCmpTotLim
  Constant7 : Constant  Value=PullCmpActvLongTermLim
  CopyRight2 : Subsystem  Description=|  mask(Copyright Information){none=on}
      | Copyright info block.                                               
      |                                                                     
      | Place copyright information at the top of every subsystem in design.
      mask prompts: none "No parameters"
      mask help: Place copyright information at the top of every subsystem in design.
      mask Display:
      | NxtrConf = 'Nexteer Confidential';
      | 
      | sys = bdroot; %handle for the current model ("system")
      | first = get_param(sys,'Created');
      | if(isempty(first))
      |     first = datestr(now,'yyyy');
      | else
      |     first = first(end-3:end);  %year is last four digits
      | end
      | 
      | last = get_param(sys,'LastModifiedDate');
      | if isempty(last)
      |     last = datestr(now,'yyyy');
      | else
      |     last = last(end-3:end);
      | end
      | 
      | if strcmp(first,last)
      |     fprintf('%s -- Copyright %s Nexteer',NxtrConf,first)
      | else
      |     fprintf('%s -- %s%s- %s Nexteer',NxtrConf,char(169),first,last)
      | end
  Data Store Read2 : DataStoreRead  DataStoreName=CmpLrnTiLongTerm
  If : If  IfExpression=u1
  If Action Subsystem : Subsystem  TreatAsAtomicUnit=on
  If Action Subsystem1 : Subsystem  TreatAsAtomicUnit=on
  LimDyn_f1 : NxtrLim/LimDyn_f32
  LimDyn_f32 : NxtrLim/LimDyn_f32
  Max_f32 : NxtrMax/Max_f32  SFunctionSpec=single y1 = Max_f32(single u1, single u2)
      settings: AttributesFormatString=%<Name>
  Merge : Merge
  Min_f1 : NxtrMin/Min_f32  SFunctionSpec=single y1 = Min_f32(single u1, single u2)
      settings: AttributesFormatString=%<Name>
  Product : Product
  Relational Operator1 : RelationalOperator  OutDataTypeStr=boolean
  Subtract : Sum
  Subtract1 : Sum  Inputs=+-
  Unary Minus : UnaryMinus
  Unary Minus1 : UnaryMinus
  Unary Minus2 : UnaryMinus
  CmpLongTerm : Outport
  wires:
  PullErrLongTerm/1 -> LimDyn_f1/1
  LimDyn_f1/1 -> Product/1
  Merge/1 -> Product/2
  Product/1 -> Subtract/2  "LongTermErrTerm"
  CmpLongTermPrev/1 -> Subtract/1
  Subtract/1 -> LimDyn_f32/1
  Constant6/1 -> Min_f1/1
  Constant5/1 -> Unary Minus/1
  Unary Minus/1 -> Max_f32/1
  Max_f32/1 -> LimDyn_f32/2
  Constant4/1 -> Min_f1/2
  Constant7/1 -> Unary Minus1/1
  Unary Minus1/1 -> Max_f32/2
  Min_f1/1 -> LimDyn_f32/3
  LimDyn_f32/1 -> CmpLongTerm/1
  Constant/1 -> Unary Minus2/1, LimDyn_f1/3
  Unary Minus2/1 -> LimDyn_f1/2
  If/2 -> If Action Subsystem1/Action
  If/1 -> If Action Subsystem/Action
  If Action Subsystem/1(LrnTiLongTerm) -> Merge/1
  If Action Subsystem1/1(LrnTiLongTerm) -> Merge/2
  Data Store Read2/1 -> Subtract1/2, If Action Subsystem1/1(In1)
  Constant1/1 -> Subtract1/1, If Action Subsystem/1(In2)
  Relational Operator1/1 -> If/1
  Constant2/1 -> Relational Operator1/2
  Subtract1/1 -> Relational Operator1/1

== system SF013A_PullCmpActv/PullCmpActv/PullCmpActvPer1/PullCmpActvPer1/ActvCmpEna/ElapsedTime/If not true elapsed time = 0 ==
  Action Port : ActionPort  ActionType=then
  Constant : Constant  Value=0  OutDataTypeStr=single
  SpanTi : Outport
  wires:
  Constant/1 -> SpanTi/1

== system SF013A_PullCmpActv/PullCmpActv/PullCmpActvPer1/PullCmpActvPer1/ActvCmpEna/ElapsedTime/If true and last step is true calculate elapsed time  ==
  Action Port : ActionPort  ActionType=else
  Constant1 : Constant  Value=MICROSECTOSEC_ULS_F32
  Data Store Read : DataStoreRead  DataStoreName=RefTiEnaLrng
  Divide : Product  Inputs=**
  FixdToFloat_f32_u32 : FixdToFloat/FixdToFloat_f32_u32  Param1=0
  GetTiSpan100MicroSec32bit : Subsystem
  SpanTi : Outport
  wires:
  Constant1/1 -> Divide/2
  Divide/1 -> SpanTi/1
  GetTiSpan100MicroSec32bit/1(TiSpan) -> FixdToFloat_f32_u32/1
  Data Store Read/1 -> GetTiSpan100MicroSec32bit/1(RefTmr)
  FixdToFloat_f32_u32/1 -> Divide/1

== system SF013A_PullCmpActv/PullCmpActv/PullCmpActvPer1/PullCmpActvPer1/ActvCmpEna/ElapsedTime/If true and last step not true elapsed time = 0 get reference time  ==
  Action Port : ActionPort  ActionType=elseif
  Constant : Constant  Value=0  OutDataTypeStr=single
  Data Store Write : DataStoreWrite  DataStoreName=RefTiEnaLrng
  GetRefTmr100MicroSec32bit : Subsystem
  "SpanTi " : Outport
  wires:
  Constant/1 -> "SpanTi "/1
  GetRefTmr100MicroSec32bit/1(RefTmr) -> Data Store Write/1

== system SF013A_PullCmpActv/PullCmpActv/PullCmpActvPer1/PullCmpActvPer1/Calc_CmpTot/If Action Subsystem/CopyRight2 ==

== system SF013A_PullCmpActv/PullCmpActv/PullCmpActvPer1/PullCmpActvPer1/Calc_CmpTot/If Action Subsystem1/CopyRight2 ==

== system SF013A_PullCmpActv/PullCmpActv/PullCmpActvPer1/PullCmpActvPer1/ShoTermCmp/CalcIntgtrGain /CopyRight2 ==

== system SF013A_PullCmpActv/PullCmpActv/PullCmpActvPer1/PullCmpActvPer1/ShoTermCmp/CalcIntgtrGain /ElapsedTime ==
  note: If
  "OpstSign " : Inport
  CopyRight2 : Subsystem  Description=|  mask(Copyright Information){none=on}
      | Copyright info block.                                               
      |                                                                     
      | Place copyright information at the top of every subsystem in design.
      mask prompts: none "No parameters"
      mask help: Place copyright information at the top of every subsystem in design.
      mask Display:
      | NxtrConf = 'Nexteer Confidential';
      | 
      | sys = bdroot; %handle for the current model ("system")
      | first = get_param(sys,'Created');
      | if(isempty(first))
      |     first = datestr(now,'yyyy');
      | else
      |     first = first(end-3:end);  %year is last four digits
      | end
      | 
      | last = get_param(sys,'LastModifiedDate');
      | if isempty(last)
      |     last = datestr(now,'yyyy');
      | else
      |     last = last(end-3:end);
      | end
      | 
      | if strcmp(first,last)
      |     fprintf('%s -- Copyright %s Nexteer',NxtrConf,first)
      | else
      |     fprintf('%s -- %s%s- %s Nexteer',NxtrConf,char(169),first,last)
      | end
  Data Store Read : DataStoreRead  Priority=1  DataStoreName=OpstSignPrev
      settings: AttributesFormatString=priority: %<Priority>
  Data Store Write : DataStoreWrite  Priority=2  DataStoreName=OpstSignPrev
      settings: AttributesFormatString="priority:  %<Priority>"
  If : If  NumInputs=2  IfExpression=u1  ElseIfExpressions=u2
  If not true elapsed time = 0 : Subsystem  TreatAsAtomicUnit=on
  "If true and last step is true calculate elapsed time " : Subsystem  TreatAsAtomicUnit=on
  "If true and last step not true elapsed time = 0 get reference time " : Subsystem  TreatAsAtomicUnit=on
  Logical Operator : Logic  AllPortsSameDT=off  OutDataTypeStr=boolean
  Logical Operator1 : Logic  Operator=NOT  AllPortsSameDT=off  OutDataTypeStr=boolean
  Logical Operator2 : Logic  Operator=NOT  AllPortsSameDT=off  OutDataTypeStr=boolean
  Merge : Merge  Inputs=3
  ElapsedTime : Outport
  wires:
  If/1 -> If not true elapsed time = 0/Action
  If/2 -> "If true and last step not true elapsed time = 0 get reference time "/Action
  If/3 -> "If true and last step is true calculate elapsed time "/Action
  If not true elapsed time = 0/1(SpanTi) -> Merge/1
  "If true and last step not true elapsed time = 0 get reference time "/1("SpanTi ") -> Merge/2
  "If true and last step is true calculate elapsed time "/1(SpanTi) -> Merge/3
  Merge/1 -> ElapsedTime/1
  "OpstSign "/1 -> Logical Operator2/1, Logical Operator/1, Data Store Write/1
  Logical Operator1/1 -> Logical Operator/2
  Data Store Read/1 -> Logical Operator1/1
  Logical Operator/1 -> If/2
  Logical Operator2/1 -> If/1

== system SF013A_PullCmpActv/PullCmpActv/PullCmpActvPer1/PullCmpActvPer1/ShoTermCmp/CalcIntgtrGain /If Action Subsystem ==
  In1 : Inport
  Action Port : ActionPort  ActionType=then
  CopyRight2 : Subsystem  Description=|  mask(Copyright Information){none=on}
      | Copyright info block.                                               
      |                                                                     
      | Place copyright information at the top of every subsystem in design.
      mask prompts: none "No parameters"
      mask help: Place copyright information at the top of every subsystem in design.
      mask Display:
      | NxtrConf = 'Nexteer Confidential';
      | 
      | sys = bdroot; %handle for the current model ("system")
      | first = get_param(sys,'Created');
      | if(isempty(first))
      |     first = datestr(now,'yyyy');
      | else
      |     first = first(end-3:end);  %year is last four digits
      | end
      | 
      | last = get_param(sys,'LastModifiedDate');
      | if isempty(last)
      |     last = datestr(now,'yyyy');
      | else
      |     last = last(end-3:end);
      | end
      | 
      | if strcmp(first,last)
      |     fprintf('%s -- Copyright %s Nexteer',NxtrConf,first)
      | else
      |     fprintf('%s -- %s%s- %s Nexteer',NxtrConf,char(169),first,last)
      | end
  Out1 : Outport
  wires:
  In1/1 -> Out1/1

== system SF013A_PullCmpActv/PullCmpActv/PullCmpActvPer1/PullCmpActvPer1/ShoTermCmp/CalcIntgtrGain /If Action Subsystem1 ==
  In1 : Inport
  Action Port : ActionPort  ActionType=else
  CopyRight2 : Subsystem  Description=|  mask(Copyright Information){none=on}
      | Copyright info block.                                               
      |                                                                     
      | Place copyright information at the top of every subsystem in design.
      mask prompts: none "No parameters"
      mask help: Place copyright information at the top of every subsystem in design.
      mask Display:
      | NxtrConf = 'Nexteer Confidential';
      | 
      | sys = bdroot; %handle for the current model ("system")
      | first = get_param(sys,'Created');
      | if(isempty(first))
      |     first = datestr(now,'yyyy');
      | else
      |     first = first(end-3:end);  %year is last four digits
      | end
      | 
      | last = get_param(sys,'LastModifiedDate');
      | if isempty(last)
      |     last = datestr(now,'yyyy');
      | else
      |     last = last(end-3:end);
      | end
      | 
      | if strcmp(first,last)
      |     fprintf('%s -- Copyright %s Nexteer',NxtrConf,first)
      | else
      |     fprintf('%s -- %s%s- %s Nexteer',NxtrConf,char(169),first,last)
      | end
  Out1 : Outport
  wires:
  In1/1 -> Out1/1

== system SF013A_PullCmpActv/PullCmpActv/PullCmpActvPer1/PullCmpActvPer1/ShoTermCmp/CalcIntgtrGain /If Action Subsystem2 ==
  CmpLrnTi_Dec_ShoTerm : Inport
  Action Port : ActionPort  ActionType=then
  Constant3 : Constant  Value=INTGTRSCARSHOTERM_ULS_F32
  Constant4 : Constant  Value=ARCHGLBPRM_2MILLISEC_SEC_F32
  CopyRight2 : Subsystem  Description=|  mask(Copyright Information){none=on}
      | Copyright info block.                                               
      |                                                                     
      | Place copyright information at the top of every subsystem in design.
      mask prompts: none "No parameters"
      mask help: Place copyright information at the top of every subsystem in design.
      mask Display:
      | NxtrConf = 'Nexteer Confidential';
      | 
      | sys = bdroot; %handle for the current model ("system")
      | first = get_param(sys,'Created');
      | if(isempty(first))
      |     first = datestr(now,'yyyy');
      | else
      |     first = first(end-3:end);  %year is last four digits
      | end
      | 
      | last = get_param(sys,'LastModifiedDate');
      | if isempty(last)
      |     last = datestr(now,'yyyy');
      | else
      |     last = last(end-3:end);
      | end
      | 
      | if strcmp(first,last)
      |     fprintf('%s -- Copyright %s Nexteer',NxtrConf,first)
      | else
      |     fprintf('%s -- %s%s- %s Nexteer',NxtrConf,char(169),first,last)
      | end
  Data Store Write : DataStoreWrite  DataStoreName=IntgtrGainDecShoTerm
  Data Store Write1 : DataStoreWrite  DataStoreName=CmpLrnTiDecShoTerm
  Divide : Product  Inputs=*/
  Product : Product
  CmpIntglGain_Dec_ShoTerm : Outport
  wires:
  Constant3/1 -> Divide/1
  Product/1 -> CmpIntglGain_Dec_ShoTerm/1, Data Store Write/1
  Constant4/1 -> Product/1
  Divide/1 -> Product/2
  CmpLrnTi_Dec_ShoTerm/1 -> Data Store Write1/1, Divide/2
